simulink model "fleet_model"  (R2014a)
settings: Solver=ode45  StartTime=0.0  StopTime=run_time  RelTol=1e-3
values from neighbouring files (symbols this model uses):
  lin_v_1 = 1    [initialization.m]
  Sample_Time = 0.05    [gmm_estimate_V1.m]    (also in gmm_estimate_V2.m; gmm_estimate_V3.m; initialization.m)
  theta0 = 0*pi/180    (= 0)    [initialization.m]
  y1_0 = y1_d    (= 250)    [initialization.m]
  y1_d = 250    [initialization.m]
  y2_0 = 220    [initialization.m]
  y3_0 = 290    [initialization.m]
  y_left_most = 1    [initialization.m]
  y_right_most = 500    [initialization.m]
libraries: dspsrcs4 x3
settings Model: Creator=User  LastModifiedBy=meinf12001
settings DataIOCC: LimitDataPoints=off

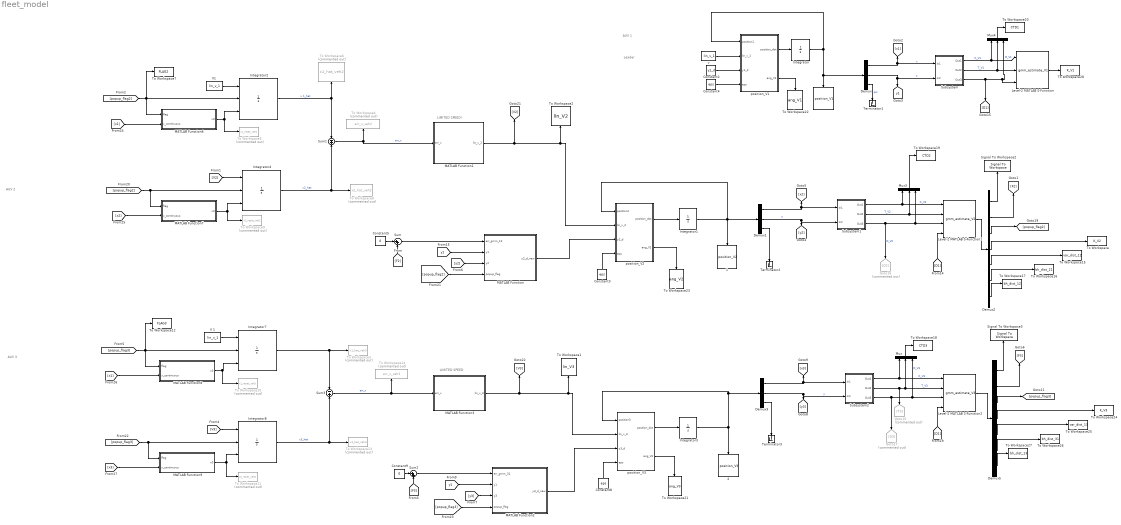
== system fleet_model ==
  note: Leader
  note: LIMITED SPEED
  note: LIMITED SPEED!
  note: AUV 1
  note: AUV 2
  note: AUV 3
  " " : ToWorkspace  VariableName=position_V1  SampleTime=Sample_Time
  " 1" : ToWorkspace  VariableName=position_V2  SampleTime=Sample_Time
  " 2" : ToWorkspace  VariableName=position_V3  SampleTime=Sample_Time
  Constant2 : Constant  Value=y1_d  SampleTime=Sample_Time
  Constant3 : Constant  Value=eps  SampleTime=Sample_Time
  Constant4 : Constant  Value=eps  SampleTime=Sample_Time
  Constant5 : Constant  Value=0  SampleTime=Sample_Time
  Constant8 : Constant  Value=eps  SampleTime=Sample_Time
  Constant9 : Constant  Value=0  SampleTime=Sample_Time
  Demux : Demux  Outputs=3
  Demux1 : Demux  Outputs=3
  Demux2 : Demux  Outputs=7
  Demux3 : Demux  Outputs=3
  Demux5 : Demux  Outputs=7
  Goto10 : Goto  Commented=on  GotoTag=T3
  Goto16 : Goto  Commented=on  GotoTag=D2
  Goto17 : Goto  Commented=on  GotoTag=D3
  Integrator : Integrator  InitialCondition=[0;y1_0;theta0]
  Integrator1 : Integrator  InitialCondition=[0;y2_0;theta0]
  Integrator{2,4,7..8} (4 alike) : Integrator  ExternalReset=level hold  InitialConditionSource=external
  Integrator3 : Integrator  InitialCondition=[0;y3_0;theta0]
  Level-2 MATLAB S-Function : M-S-Function  FunctionName=gmm_estimate_V1
  Level-2 MATLAB S-Function1 : M-S-Function  FunctionName=gmm_estimate_V2
  Level-2 MATLAB S-Function2 : M-S-Function  FunctionName=gmm_estimate_V3
  MATLAB Function : MATLAB Function  TreatAsAtomicUnit=on
  MATLAB Function1 : MATLAB Function  TreatAsAtomicUnit=on
  MATLAB Function2 : MATLAB Function  TreatAsAtomicUnit=on
  MATLAB Function3 : MATLAB Function  TreatAsAtomicUnit=on
  MATLAB Function6 : MATLAB Function  TreatAsAtomicUnit=on
  MATLAB Function7 : MATLAB Function  TreatAsAtomicUnit=on
  MATLAB Function8 : MATLAB Function  TreatAsAtomicUnit=on
  MATLAB Function9 : MATLAB Function  TreatAsAtomicUnit=on
  Mux : Mux  Inputs=3
  Mux3 : Mux  Inputs=3
  Mux4 : Mux  Inputs=3
  Signal To Workspace2 : SignalToWorkspace  VariableName=err_gmm_12
      settings: CopyFcn=dspblkcopystw(gcbh);  Save2DSignal=Inherit from input (this choice will be removed - see release notes)
  Signal To Workspace3 : SignalToWorkspace  VariableName=err_gmm_31
      settings: CopyFcn=dspblkcopystw(gcbh);  Save2DSignal=Inherit from input (this choice will be removed - see release notes)
  Subsystem : Subsystem
  Subsystem1 : Subsystem
  Subsystem2 : Subsystem
  Sum : Sum  Inputs=|++
  Sum1 : Sum  Inputs=-|+
  Sum2 : Sum  Inputs=|++
  Sum3 : Sum  Inputs=-|+
  Terminator1 : Terminator
  Terminator2 : Terminator
  Terminator3 : Terminator
  To Workspace : ToWorkspace  VariableName=K_V2  SampleTime=Sample_Time
  To Workspace1 : ToWorkspace  VariableName=lin_V3  SampleTime=Sample_Time
  To Workspace10 : ToWorkspace  Commented=on  VariableName=x1_reset_veh3  SampleTime=-1
  To Workspace11 : ToWorkspace  Commented=on  VariableName=x3_reset_veh3  SampleTime=-1
  To Workspace12 : ToWorkspace  VariableName=FLAG3  SampleTime=Sample_Time
  To Workspace13 : ToWorkspace  Commented=on  VariableName=x3_hat_veh3  SampleTime=-1
  To Workspace14 : ToWorkspace  Commented=on  VariableName=err_x_veh3  SampleTime=-1
  To Workspace15 : ToWorkspace  VariableName=var_dist_12  SampleTime=Sample_Time
  To Workspace16 : ToWorkspace  VariableName=bh_dist_21  SampleTime=Sample_Time
  To Workspace17 : ToWorkspace  VariableName=bh_dist_12  SampleTime=Sample_Time
  To Workspace18 : ToWorkspace  VariableName=CTD3  SampleTime=Sample_Time
  To Workspace19 : ToWorkspace  VariableName=CTD2  SampleTime=Sample_Time
  To Workspace2 : ToWorkspace  VariableName=lin_V2  SampleTime=Sample_Time
  To Workspace20 : ToWorkspace  VariableName=CTD1  SampleTime=Sample_Time
  To Workspace21 : ToWorkspace  VariableName=ang_V3  SampleTime=Sample_Time
  To Workspace22 : ToWorkspace  VariableName=ang_V1  SampleTime=Sample_Time
  To Workspace23 : ToWorkspace  VariableName=ang_V2  SampleTime=Sample_Time
  To Workspace24 : ToWorkspace  VariableName=K_V3  SampleTime=Sample_Time
  To Workspace25 : ToWorkspace  VariableName=var_dist_13  SampleTime=Sample_Time
  To Workspace26 : ToWorkspace  VariableName=bh_dist_31  SampleTime=Sample_Time
  To Workspace27 : ToWorkspace  VariableName=bh_dist_13  SampleTime=Sample_Time
  To Workspace28 : ToWorkspace  VariableName=K_V1  SampleTime=Sample_Time
  To Workspace3 : ToWorkspace  Commented=on  VariableName=x1_hat_veh3  SampleTime=-1
  To Workspace4 : ToWorkspace  Commented=on  VariableName=err_x_veh2  SampleTime=-1
  To Workspace5 : ToWorkspace  Commented=on  VariableName=x1_reset_veh2  SampleTime=-1
  To Workspace6 : ToWorkspace  Commented=on  VariableName=x1_hat_veh2  SampleTime=-1
  To Workspace7 : ToWorkspace  VariableName=FLAG2  SampleTime=Sample_Time
  To Workspace8 : ToWorkspace  Commented=on  VariableName=x2_hat_veh2  SampleTime=-1
  To Workspace9 : ToWorkspace  Commented=on  VariableName=x2_reset_veh2  SampleTime=-1
  V 1 : Constant  Value=lin_v_1  SampleTime=Sample_Time
  V1 : Constant  Value=lin_v_1  SampleTime=Sample_Time
  "position_V1 " : MATLAB Function  TreatAsAtomicUnit=on
  "position_V2 " : MATLAB Function  TreatAsAtomicUnit=on
  "position_V3 " : MATLAB Function  TreatAsAtomicUnit=on
  v : Constant  Value=lin_v_1  SampleTime=Sample_Time
  tag scope: y1=global
  wires:
  Demux/1 -> Subsystem/1(In1), [x1]  "x"
  Demux/2 -> Subsystem/2(In2), [y1]  "y"
  Integrator/1 -> Demux/1, " "/1, "position_V1 "/1(position1)
  "position_V1 "/1(position_dot) -> Integrator/1
  Demux/3 -> Terminator1/1  "psi"
  Integrator1/1 -> " 1"/1, "position_V2 "/1(position2), Demux1/1
  "position_V2 "/1(position_dot) -> Integrator1/1
  Demux1/3 -> Terminator2/1
  Subsystem1/1(Out1) -> Mux3/1, Level-2 MATLAB S-Function1/1  "C_V2"
  Subsystem1/2(Out2) -> Level-2 MATLAB S-Function1/2, Mux3/2  "T_V2"
  Subsystem1/3(Out3) -> Level-2 MATLAB S-Function1/3, Mux3/3, Goto16/1  "D_V2"
  Demux1/1 -> Subsystem1/1(In1), [x2]
  Demux1/2 -> Subsystem1/2(In2), [y2]  "y"
  Constant2/1 -> "position_V1 "/3(y1_d)
  v/1 -> "position_V1 "/2(lin_v_1)
  Constant4/1 -> "position_V1 "/4(eps)
  Constant3/1 -> "position_V2 "/4(eps)
  Subsystem/1(Out1) -> Mux4/1, Level-2 MATLAB S-Function/1  "C_V1"
  Subsystem/2(Out2) -> Level-2 MATLAB S-Function/2, Mux4/2  "T_V1"
  Subsystem/3(Out3) -> Level-2 MATLAB S-Function/3, Mux4/3, [D1]  "D_V1"
  Level-2 MATLAB S-Function1/1 -> Demux2/1
  Demux2/1 -> Signal To Workspace2/1
  Demux2/2 -> [F2]
  MATLAB Function/1(y2_d_new) -> "position_V2 "/3(y2_d)
  Sum/1 -> MATLAB Function/1(err_gmm_12)
  Constant5/1 -> Sum/1
  [F2] -> Sum/2
  Integrator2/1 -> Sum1/1, To Workspace6/1  "x 1_hat"
  Sum1/1 -> To Workspace4/1, MATLAB Function1/1(err_x)  "err_x"
  [y2] -> MATLAB Function/3(y2)
  Integrator3/1 -> " 2"/1, Demux3/1, "position_V3 "/1(position3)
  "position_V3 "/1(position_dot) -> Integrator3/1
  Demux3/3 -> Terminator3/1
  Subsystem2/1(Out1) -> Mux/1, Level-2 MATLAB S-Function2/1  "C_V3"
  Subsystem2/2(Out2) -> Goto10/1, Level-2 MATLAB S-Function2/2, Mux/2  "T_V3"
  Subsystem2/3(Out3) -> Mux/3, Level-2 MATLAB S-Function2/3, Goto17/1  "D_V3"
  Demux3/1 -> Subsystem2/1(In1), [x3]
  Demux3/2 -> Subsystem2/2(In2), [y3]  "y"
  Constant8/1 -> "position_V3 "/4(eps)
  Level-2 MATLAB S-Function2/1 -> Demux5/1
  MATLAB Function2/1(y3_d_new) -> "position_V3 "/3(y3_d)
  Sum2/1 -> MATLAB Function2/1(err_gmm_31)
  Constant9/1 -> Sum2/1
  [F3] -> Sum2/2
  [y3] -> MATLAB Function2/3(y3)
  Demux2/3 -> [popup_flag2]
  [D1] -> Level-2 MATLAB S-Function1/4
  [D1] -> Level-2 MATLAB S-Function2/4
  [popup_flag2] -> MATLAB Function/4(popup_flag)
  [popup_flag3] -> MATLAB Function2/4(popup_flag)
  MATLAB Function1/1(lin_v_2) -> [V2], "position_V2 "/2(lin_v_2), To Workspace2/1
  MATLAB Function3/1(lin_v_3) -> [V3], "position_V3 "/2(lin_v_3), To Workspace1/1
  V1/1 -> Integrator2/1
  MATLAB Function6/1(x0) -> To Workspace5/1, Integrator2/3
  [popup_flag2] -> To Workspace7/1, MATLAB Function6/1(flag), Integrator2/2
  [x1] -> MATLAB Function6/2(x_continuous)
  Integrator4/1 -> Sum1/2, To Workspace8/1  "x2_hat"
  [V2] -> Integrator4/1
  MATLAB Function7/1(x0) -> To Workspace9/1, Integrator4/3
  [popup_flag2] -> Integrator4/2, MATLAB Function7/1(flag)
  [x2] -> MATLAB Function7/2(x_continuous)
  Sum3/1 -> MATLAB Function3/1(err_x), To Workspace14/1  "err_x"
  V 1/1 -> Integrator7/1
  MATLAB Function8/1(x0) -> To Workspace10/1, Integrator7/3
  [popup_flag3] -> To Workspace12/1, Integrator7/2, MATLAB Function8/1(flag)
  [x1] -> MATLAB Function8/2(x_continuous)
  Integrator8/1 -> Sum3/2, To Workspace13/1  "x3_hat"
  [V3] -> Integrator8/1
  MATLAB Function9/1(x0) -> To Workspace11/1, Integrator8/3
  [popup_flag3] -> MATLAB Function9/1(flag), Integrator8/2
  [x3] -> MATLAB Function9/2(x_continuous)
  Integrator7/1 -> Sum3/1, To Workspace3/1
  Mux/1 -> To Workspace18/1
  Mux3/1 -> To Workspace19/1
  Mux4/1 -> To Workspace20/1
  "position_V3 "/2(ang_V3) -> To Workspace21/1
  "position_V2 "/2(ang_V2) -> To Workspace23/1
  "position_V1 "/2(ang_V1) -> To Workspace22/1
  [y1] -> MATLAB Function2/2(y1)
  [y1] -> MATLAB Function/2(y1)
  Demux2/4 -> To Workspace/1
  Demux2/5 -> To Workspace15/1
  Demux2/6 -> To Workspace16/1
  Demux2/7 -> To Workspace17/1
  Demux5/1 -> Signal To Workspace3/1
  Demux5/2 -> [F3]
  Demux5/3 -> [popup_flag3]
  Demux5/4 -> To Workspace24/1
  Demux5/5 -> To Workspace25/1
  Demux5/6 -> To Workspace26/1
  Demux5/7 -> To Workspace27/1
  Level-2 MATLAB S-Function/1 -> To Workspace28/1

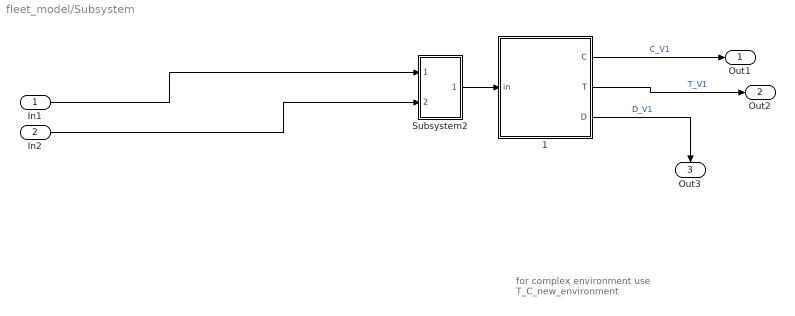
== system fleet_model/Subsystem ==
  note: for complex environment use
      | T_C_new_environment
  In1 : Inport
  In2 : Inport  Port=2
  " 1" : MATLAB Function  TreatAsAtomicUnit=on
  Subsystem2 : Subsystem
  Out1 : Outport
  Out2 : Outport  Port=2
  Out3 : Outport  Port=3
  wires:
  " 1"/2(T) -> Out2/1  "T_V1"
  " 1"/3(D) -> Out3/1  "D_V1"
  " 1"/1(C) -> Out1/1  "C_V1"
  In1/1 -> Subsystem2/1(In1)
  In2/1 -> Subsystem2/2(In2)
  Subsystem2/1(Out1) -> " 1"/1(in)

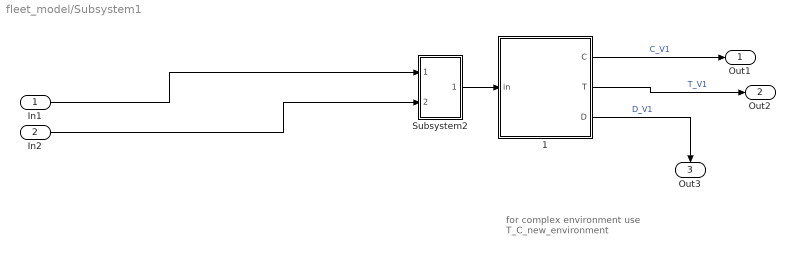
== system fleet_model/Subsystem1 ==
  note: for complex environment use
      | T_C_new_environment
  In1 : Inport
  In2 : Inport  Port=2
  " 1" : MATLAB Function  TreatAsAtomicUnit=on
  Subsystem2 : Subsystem
  Out1 : Outport
  Out2 : Outport  Port=2
  Out3 : Outport  Port=3
  wires:
  " 1"/2(T) -> Out2/1  "T_V1"
  " 1"/3(D) -> Out3/1  "D_V1"
  " 1"/1(C) -> Out1/1  "C_V1"
  In1/1 -> Subsystem2/1(In1)
  In2/1 -> Subsystem2/2(In2)
  Subsystem2/1(Out1) -> " 1"/1(in)

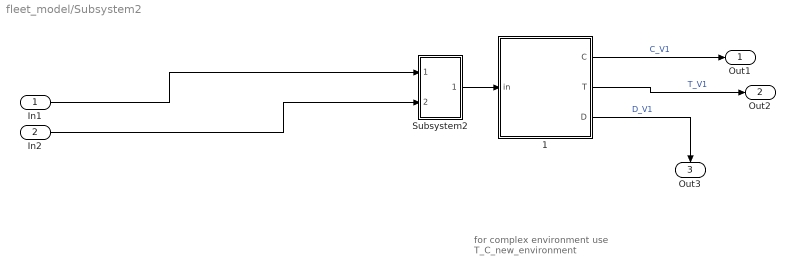
== system fleet_model/Subsystem2 ==
  note: for complex environment use
      | T_C_new_environment
  In1 : Inport
  In2 : Inport  Port=2
  " 1" : MATLAB Function  TreatAsAtomicUnit=on
  Subsystem2 : Subsystem
  Out1 : Outport
  Out2 : Outport  Port=2
  Out3 : Outport  Port=3
  wires:
  " 1"/2(T) -> Out2/1  "T_V1"
  " 1"/3(D) -> Out3/1  "D_V1"
  " 1"/1(C) -> Out1/1  "C_V1"
  In1/1 -> Subsystem2/1(In1)
  In2/1 -> Subsystem2/2(In2)
  Subsystem2/1(Out1) -> " 1"/1(in)

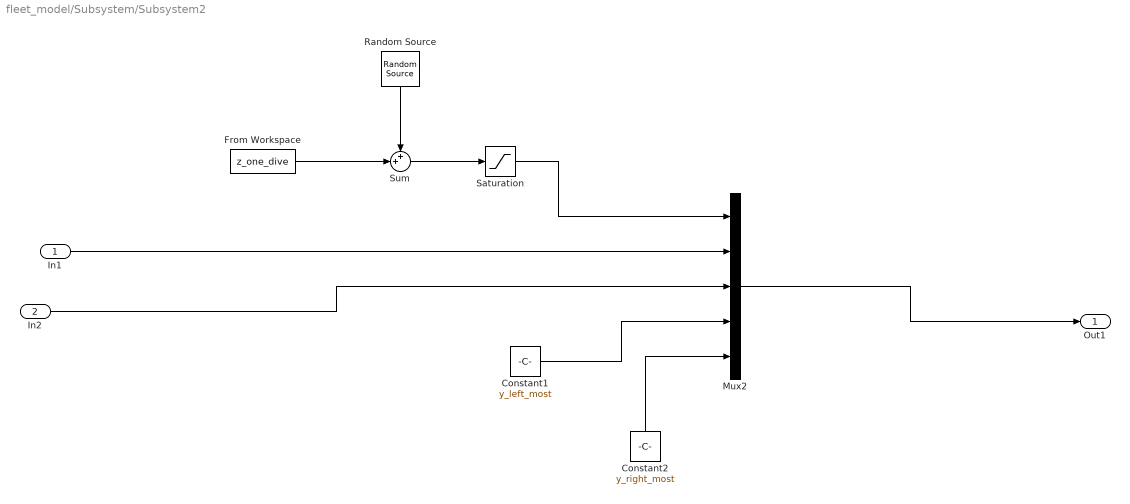
== system fleet_model/Subsystem/Subsystem2 ==
  In1 : Inport
  In2 : Inport  Port=2
  Constant1 : Constant  Value=y_left_most  SampleTime=Sample_Time
  Constant2 : Constant  Value=y_right_most  SampleTime=Sample_Time
  From Workspace : FromWorkspace  VariableName=z_one_dive  SampleTime=Sample_Time  Interpolate=off  OutputAfterFinalValue=Cyclic repetition
  Mux2 : Mux  Inputs=5
  Random Source : dspsrcs4/Random Source  SrcType=Gaussian  NormMethod=Ziggurat  CltLength=12  MinVal=0  MaxVal=1  MeanVal=0  VarVal=.001  RepMode=Repeatable  rawSeed=1  IsInherit=on  SampMode=Continuous  SampTime=1  SampFrame=1  DataType=Single  OutComplex=Real
  Saturation : Saturate  UpperLimit=1  LowerLimit=0  ZeroCross=off
  Sum : Sum  Inputs=++|
  Out1 : Outport
  wires:
  In1/1 -> Mux2/2
  Constant2/1 -> Mux2/5
  Constant1/1 -> Mux2/4
  Mux2/1 -> Out1/1
  In2/1 -> Mux2/3
  Sum/1 -> Saturation/1
  From Workspace/1 -> Sum/2
  Random Source/1 -> Sum/1
  Saturation/1 -> Mux2/1

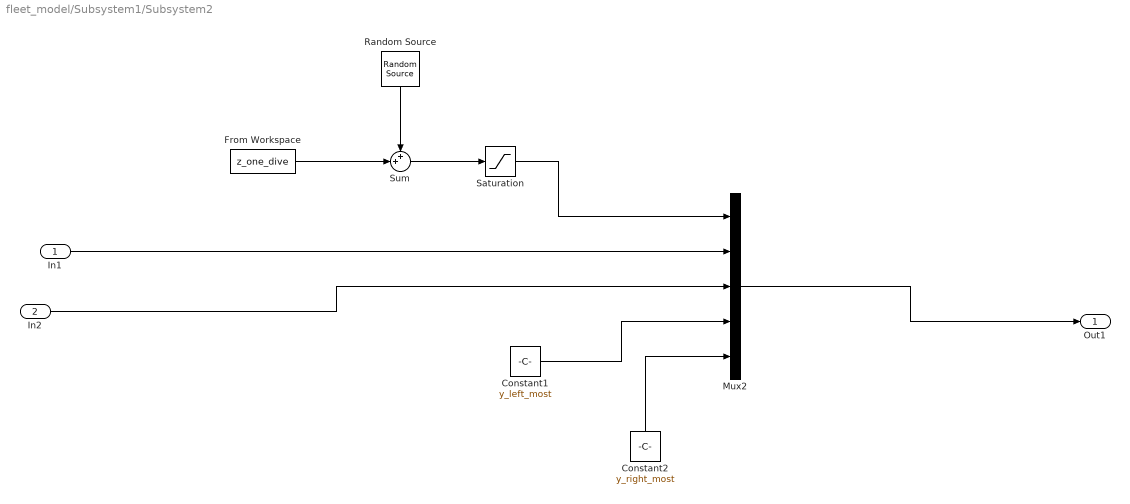
== system fleet_model/Subsystem1/Subsystem2 ==
  In1 : Inport
  In2 : Inport  Port=2
  Constant1 : Constant  Value=y_left_most  SampleTime=Sample_Time
  Constant2 : Constant  Value=y_right_most  SampleTime=Sample_Time
  From Workspace : FromWorkspace  VariableName=z_one_dive  SampleTime=Sample_Time  Interpolate=off  OutputAfterFinalValue=Cyclic repetition
  Mux2 : Mux  Inputs=5
  Random Source : dspsrcs4/Random Source  SrcType=Gaussian  NormMethod=Ziggurat  CltLength=12  MinVal=0  MaxVal=1  MeanVal=0  VarVal=.001  RepMode=Repeatable  rawSeed=1  IsInherit=on  SampMode=Continuous  SampTime=1  SampFrame=1  DataType=Single  OutComplex=Real
  Saturation : Saturate  UpperLimit=1  LowerLimit=0  ZeroCross=off
  Sum : Sum  Inputs=++|
  Out1 : Outport
  wires:
  In1/1 -> Mux2/2
  Constant2/1 -> Mux2/5
  Constant1/1 -> Mux2/4
  Mux2/1 -> Out1/1
  In2/1 -> Mux2/3
  Sum/1 -> Saturation/1
  From Workspace/1 -> Sum/2
  Random Source/1 -> Sum/1
  Saturation/1 -> Mux2/1

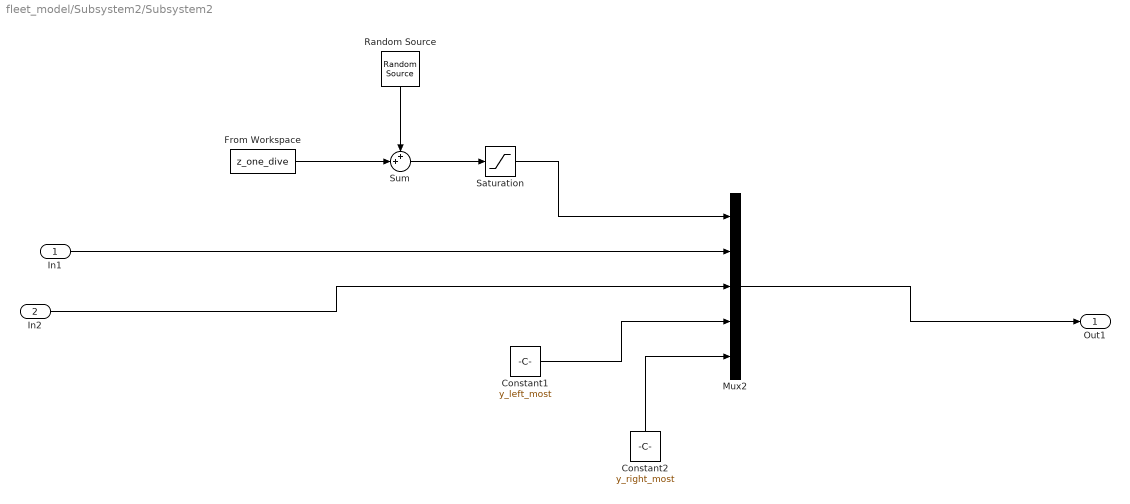
== system fleet_model/Subsystem2/Subsystem2 ==
  In1 : Inport
  In2 : Inport  Port=2
  Constant1 : Constant  Value=y_left_most  SampleTime=Sample_Time
  Constant2 : Constant  Value=y_right_most  SampleTime=Sample_Time
  From Workspace : FromWorkspace  VariableName=z_one_dive  SampleTime=Sample_Time  Interpolate=off  OutputAfterFinalValue=Cyclic repetition
  Mux2 : Mux  Inputs=5
  Random Source : dspsrcs4/Random Source  SrcType=Gaussian  NormMethod=Ziggurat  CltLength=12  MinVal=0  MaxVal=1  MeanVal=0  VarVal=.001  RepMode=Repeatable  rawSeed=1  IsInherit=on  SampMode=Continuous  SampTime=1  SampFrame=1  DataType=Single  OutComplex=Real
  Saturation : Saturate  UpperLimit=1  LowerLimit=0  ZeroCross=off
  Sum : Sum  Inputs=++|
  Out1 : Outport
  wires:
  In1/1 -> Mux2/2
  Constant2/1 -> Mux2/5
  Constant1/1 -> Mux2/4
  Mux2/1 -> Out1/1
  In2/1 -> Mux2/3
  Sum/1 -> Saturation/1
  From Workspace/1 -> Sum/2
  Random Source/1 -> Sum/1
  Saturation/1 -> Mux2/1

== matlab function fleet_model/Subsystem/ 1 ==
  data: C output; in input; T output; D output
function [C, T, D] = T_C_estimate(in)
%#codegen
% x can anything
% y [y_left_d y_right_d]
z = in(1);
x = in(2);
y = in(3);
y_left_d = in(4);
y_right_d = in(5);
D = z * 11.55 ;
y_original = y ;
y = (y - y_left_d)/(y_right_d - y_left_d) ;
% pi = 3.1415 ;
...........................................................................
% popup4 regression model
% temperature
% Coefficients (with 95% confidence bounds):
       a =       20.91  ; % (19.9, 19.91)
       b =    -0.02081  ; % (-0.02687, -0.01475)
       c =      0.2248  ; % (0.2138, 0.2358)
       m =       2.879  ; % (2.695, 3.063)
       w =       2.615  ; % (2.468, 2.763)
T_right = a + b*sin(m*pi*y*z) + c*exp(-(w*z)^2) ;
...
    % Coefficients (with 95% confidence bounds):
       a =       5.938  ; % (-2.58e+04, 2.581e+04)
       b =     -0.0162  ; % (-0.0186, -0.01379)
       c =     -0.0148  ; % (-2.58e+04, 2.58e+04)
       m =      0.8842  ; % (0.8181, 0.9504)
       w =   -0.006801  ; % (-5928, 5928)
C_right = a + b*sin(m*pi*y*z) + c*exp(-(w*z)^2) ;

...........................................................................
% popup2 regression model
        % Coefficients (with 95% confidence bounds):
% Temperature
       a =       18.35  ; % (19.24, 19.46)   19.35
       b =     0.01291  ; % (0.008128, 0.0177)
       c =      0.4754  ; % (0.3695, 0.5813)
       m =       2.851  ; % (2.641, 3.061)
       w =     -0.8884  ; % (-1.041, -0.7359)
T_left = a + b*sin(m*pi*y*z) + c*exp(-(w*z)^2) ;

...
  % Coefficients (with 95% confidence bounds):
       a =       3.813  ; % (4.763, 4.864)   4.813
       b =   -0.003453  ; % (-0.004459, -0.002447)
       c =     0.08822  ; % (0.03802, 0.1384)
       m =       1.305  ; % (1.176, 1.434)
       w =      0.6251  ; % (0.4072, 0.8429)
C_left = a + b*sin(m*pi*y*z) + c*exp(-(w*z)^2) ;



                 if y_original <= y_left_d
                     C = C_left ;
                     T = T_left ;
                 elseif y_original >= y_right_d
                     C = C_right ;
                     T = T_right ;
                 else                     
                     C = ((y_right_d - y_original)* C_left + (y_original - y_left_d)* C_right)/(y_right_d-y_left_d) ;
                     T = ((y_right_d - y_original)* T_left + (y_original - y_left_d)* T_right)/(y_right_d-y_left_d) ;
                 end

== matlab function fleet_model/position_V1  ==
  data: position1 input; lin_v_1 input; position_dot output; y1_d input; eps input; ang_V1 output
function [position_dot,ang_V1]  = find_path(position1, lin_v_1, y1_d, eps)
%#codegen

y = position1(2) ;
psi = position1(3) ;

x_dot = lin_v_1 * cos(psi) ;
y_dot = lin_v_1 * sin(psi) ;


k1 = 1 ; 
k2 = 1.5 ;

err = y - y1_d ;
u = -(1/lin_v_1) * k1 * err ;

if abs(u) < eps
    saturated_u = u ;
elseif u > eps
    saturated_u = eps ;
else
    saturated_u = -eps ;
end

psi_d = asin(saturated_u) ; % in radian
psi_tilde = psi - psi_d ;
% psi_tilde_dot = psi_dot-(psi_d_dot==0)=psi_dot=r
r = -k2 * psi_tilde ;
psi_dot = r ;

position_dot = [x_dot; y_dot; psi_dot] ;
ang_V1 = psi_dot ;

== matlab function fleet_model/Subsystem1/ 1 ==
  data: C output; in input; T output; D output
function [C, T, D] = T_C_estimate(in)
%#codegen
% x can anything
% y [y_left_d y_right_d]
z = in(1);
x = in(2);
y = in(3);
y_left_d = in(4);
y_right_d = in(5);
D = z * 11.55 ;
y_original = y ;
y = (y - y_left_d)/(y_right_d - y_left_d) ;
% pi = 3.1415 ;
...........................................................................
% popup4 regression model
% temperature
% Coefficients (with 95% confidence bounds):
       a =       20.91  ; % (19.9, 19.91)
       b =    -0.02081  ; % (-0.02687, -0.01475)
       c =      0.2248  ; % (0.2138, 0.2358)
       m =       2.879  ; % (2.695, 3.063)
       w =       2.615  ; % (2.468, 2.763)
T_right = a + b*sin(m*pi*y*z) + c*exp(-(w*z)^2) ;
...
    % Coefficients (with 95% confidence bounds):
       a =       5.938  ; % (-2.58e+04, 2.581e+04)
       b =     -0.0162  ; % (-0.0186, -0.01379)
       c =     -0.0148  ; % (-2.58e+04, 2.58e+04)
       m =      0.8842  ; % (0.8181, 0.9504)
       w =   -0.006801  ; % (-5928, 5928)
C_right = a + b*sin(m*pi*y*z) + c*exp(-(w*z)^2) ;

...........................................................................
% popup2 regression model
        % Coefficients (with 95% confidence bounds):
% Temperature
       a =       18.35  ; % (19.24, 19.46)   19.35
       b =     0.01291  ; % (0.008128, 0.0177)
       c =      0.4754  ; % (0.3695, 0.5813)
       m =       2.851  ; % (2.641, 3.061)
       w =     -0.8884  ; % (-1.041, -0.7359)
T_left = a + b*sin(m*pi*y*z) + c*exp(-(w*z)^2) ;

...
  % Coefficients (with 95% confidence bounds):
       a =       3.813  ; % (4.763, 4.864)   4.813
       b =   -0.003453  ; % (-0.004459, -0.002447)
       c =     0.08822  ; % (0.03802, 0.1384)
       m =       1.305  ; % (1.176, 1.434)
       w =      0.6251  ; % (0.4072, 0.8429)
C_left = a + b*sin(m*pi*y*z) + c*exp(-(w*z)^2) ;



                 if y_original <= y_left_d
                     C = C_left ;
                     T = T_left ;
                 elseif y_original >= y_right_d
                     C = C_right ;
                     T = T_right ;
                 else                     
                     C = ((y_right_d - y_original)* C_left + (y_original - y_left_d)* C_right)/(y_right_d-y_left_d) ;
                     T = ((y_right_d - y_original)* T_left + (y_original - y_left_d)* T_right)/(y_right_d-y_left_d) ;
                 end

== matlab function fleet_model/position_V2  ==
  data: position2 input; lin_v_2 input; y2_d input; position_dot output; eps input; ang_V2 output
function [position_dot,ang_V2]  = find_path(position2, lin_v_2,y2_d, eps)
%#codegen

y = position2(2) ;
psi = position2(3) ;

x_dot = lin_v_2 * cos(psi) ;
y_dot = lin_v_2 * sin(psi) ;


k1 = 1 ; 
k2 = 1.5 ;

err_y = y - y2_d ;
u = -(1/lin_v_2) * k1 * err_y ;
 
if abs(u) < eps
    saturated_u = u ;
elseif u > eps
    saturated_u = eps ;
else
    saturated_u = -eps ;
end

psi_d = asin(saturated_u) ; % in radian
psi_tilde = psi - psi_d ;
% psi_tilde_dot = psi_dot-(psi_d_dot==0)=psi_dot=r
r = -k2 * psi_tilde ;
psi_dot = r ;

position_dot = [x_dot; y_dot; psi_dot] ;
ang_V2 = psi_dot ;

== matlab function fleet_model/Subsystem2/ 1 ==
  data: C output; in input; T output; D output
function [C, T, D] = T_C_estimate(in)
%#codegen
% x can anything
% y [y_left_d y_right_d]
z = in(1);
x = in(2);
y = in(3);
y_left_d = in(4);
y_right_d = in(5);
D = z * 11.55 ;
y_original = y ;
y = (y - y_left_d)/(y_right_d - y_left_d) ;
% pi = 3.1415 ;
...........................................................................
% popup4 regression model
% temperature
% Coefficients (with 95% confidence bounds):
       a =       20.91  ; % (19.9, 19.91)
       b =    -0.02081  ; % (-0.02687, -0.01475)
       c =      0.2248  ; % (0.2138, 0.2358)
       m =       2.879  ; % (2.695, 3.063)
       w =       2.615  ; % (2.468, 2.763)
T_right = a + b*sin(m*pi*y*z) + c*exp(-(w*z)^2) ;
...
    % Coefficients (with 95% confidence bounds):
       a =       5.938  ; % (-2.58e+04, 2.581e+04)
       b =     -0.0162  ; % (-0.0186, -0.01379)
       c =     -0.0148  ; % (-2.58e+04, 2.58e+04)
       m =      0.8842  ; % (0.8181, 0.9504)
       w =   -0.006801  ; % (-5928, 5928)
C_right = a + b*sin(m*pi*y*z) + c*exp(-(w*z)^2) ;

...........................................................................
% popup2 regression model
        % Coefficients (with 95% confidence bounds):
% Temperature
       a =       18.35  ; % (19.24, 19.46)   19.35
       b =     0.01291  ; % (0.008128, 0.0177)
       c =      0.4754  ; % (0.3695, 0.5813)
       m =       2.851  ; % (2.641, 3.061)
       w =     -0.8884  ; % (-1.041, -0.7359)
T_left = a + b*sin(m*pi*y*z) + c*exp(-(w*z)^2) ;

...
  % Coefficients (with 95% confidence bounds):
       a =       3.813  ; % (4.763, 4.864)   4.813
       b =   -0.003453  ; % (-0.004459, -0.002447)
       c =     0.08822  ; % (0.03802, 0.1384)
       m =       1.305  ; % (1.176, 1.434)
       w =      0.6251  ; % (0.4072, 0.8429)
C_left = a + b*sin(m*pi*y*z) + c*exp(-(w*z)^2) ;



                 if y_original <= y_left_d
                     C = C_left ;
                     T = T_left ;
                 elseif y_original >= y_right_d
                     C = C_right ;
                     T = T_right ;
                 else                     
                     C = ((y_right_d - y_original)* C_left + (y_original - y_left_d)* C_right)/(y_right_d-y_left_d) ;
                     T = ((y_right_d - y_original)* T_left + (y_original - y_left_d)* T_right)/(y_right_d-y_left_d) ;
                 end

== matlab function fleet_model/MATLAB Function ==
  data: err_gmm_12 input; y1 input; y2 input; y2_d_new output; popup_flag input
function y2_d_new = fnc( err_gmm_12, y1, y2, popup_flag)
%#codegen

err_gmm_current = err_gmm_12 ;
err_gmmm_goal = 3 ; % apparently smaller one, works better!

e = (err_gmm_current - err_gmmm_goal)/err_gmmm_goal ;

% if e < 0.0001
%     e = 0 ; % To smooth the fluctuations !
% end

min_dist = 10 ;
max_dist = 300 ;
lambda = 5 ;

persistent y_d
if isempty(y_d)
    y_d = y2 ; % y1 - min_dist ;
end
    if popup_flag
        y_d = y2 + lambda * ( e ) ;
        if (y1 - y2) > max_dist
            y_d = y1 - max_dist ;
        end
        if (y1 - y2) < min_dist
            y_d = y1 - max_dist ;
        end             
    end    
% end

y2_d_new = y_d ;

== matlab function fleet_model/MATLAB Function1 ==
  data: err_x input; lin_v_2 output
function lin_v_2  = fcn( err_x)

%#codegen
% err_x = x2 - x1
k1 = 1.2 ;
% k2 = 1.5 ;

u = - k1 * err_x ;

lin_v_2 = 1 + u ;

lin_v_2 = min( lin_v_2 , 1.5 ) ; % limited speed changes

== matlab function fleet_model/MATLAB Function2 ==
  data: y3_d_new output; err_gmm_31 input; y1 input; y3 input; popup_flag input
function y3_d_new = fnc( err_gmm_31, y1, y3, popup_flag)
%#codegen

err_gmm_current = err_gmm_31 ;
err_gmmm_goal = 3.5 ; % apparently smaller one, works better!

e = (err_gmm_current - err_gmmm_goal)/err_gmmm_goal ;

% if e < 0.0001
%     e = 0 ; % To smooth the fluctuations !
% end

min_dist = 10 ;
max_dist = 300 ;
lambda = 5 ;

persistent y_d
if isempty(y_d)
    y_d = y3 ; % y1 + min_dist ;
end
    if popup_flag
        y_d = y3 - lambda * ( e ) ;
        if (y3 - y1) > max_dist
            y_d = y1 + max_dist ;
        end
        if (y3 - y1) < min_dist
            y_d = y1 + max_dist ;
        end        
    end    
% end

y3_d_new = y_d ;

== matlab function fleet_model/MATLAB Function3 ==
  data: err_x input; lin_v_3 output
function lin_v_3  = fcn( err_x)

%#codegen
% err_x = x3 - x1
k1 = 1.2 ;
% k2 = 1.5 ;

u = - k1 * err_x ;

lin_v_3 = 1 + u ;

lin_v_3 = min( lin_v_3 , 1.5 ) ; % limited speed changes

== matlab function fleet_model/position_V3  ==
  data: position3 input; lin_v_3 input; y3_d input; position_dot output; eps input; ang_V3 output
function [position_dot,ang_V3]  = find_path(position3, lin_v_3,y3_d, eps)
%#codegen

y = position3(2) ;
psi = position3(3) ;

x_dot = lin_v_3 * cos(psi) ;
y_dot = lin_v_3 * sin(psi) ;


k1 = 1 ; 
k2 = 1.5 ;

err_y = y - y3_d ;
u = -(1/lin_v_3) * k1 * err_y ;
 
if abs(u) < eps
    saturated_u = u ;
elseif u > eps
    saturated_u = eps ;
else
    saturated_u = -eps ;
end

psi_d = asin(saturated_u) ; % in radian
psi_tilde = psi - psi_d ;
% psi_tilde_dot = psi_dot-(psi_d_dot==0)=psi_dot=r
r = -k2 * psi_tilde ;
psi_dot = r ;

position_dot = [x_dot; y_dot; psi_dot] ;
ang_V3 = psi_dot ;

== matlab function fleet_model/MATLAB Function6 ==
  data: flag input; x0 output; x_continuous input

function x0 = fcn(flag,x_continuous)
%#codegen

persistent x

if isempty(x)
    x = 0 ;
else
    if flag
        x = x_continuous ;
    end
end

x0 = x ;

== matlab function fleet_model/MATLAB Function7 ==
  data: flag input; x0 output; x_continuous input

function x0 = fcn(flag,x_continuous)
%#codegen

persistent x

if isempty(x)
    x = 0 ;
else
    if flag
        x = x_continuous ;
    end
end

x0 = x ;

== matlab function fleet_model/MATLAB Function8 ==
  data: flag input; x0 output; x_continuous input

function x0 = fcn(flag,x_continuous)
%#codegen

persistent x

if isempty(x)
    x = 0 ;
else
    if flag
        x = x_continuous ;
    end
end

x0 = x ;

== matlab function fleet_model/MATLAB Function9 ==
  data: flag input; x0 output; x_continuous input

function x0 = fcn(flag,x_continuous)
%#codegen

persistent x

if isempty(x)
    x = 0 ;
else
    if flag
        x = x_continuous ;
    end
end

x0 = x ;
